simulink model "SimulinkModel_hquad_lin_roll_1stOrd"  (Simulink 7.6)
settings: Solver=ode45  StartTime=0.0  StopTime=10.0  RelTol=1e-3
values from neighbouring files (symbols this model uses):
  g = 9.8065    [kostas_malakies.mat]    (also in kostas_malakies2.mat; load_PMModel.m = 9.81; main.m; main_last.m)
  mass = 0.66    [kostas_malakies.mat]    (also in kostas_malakies2.mat; load_PMModel.m = 0.687; main_last.m)
libraries: Hqaud_model_LIB_SI x1
settings Model: Creator=andi  LastModifiedBy=burrimi
settings DebuggingCC: StrictBusMsg=Warning

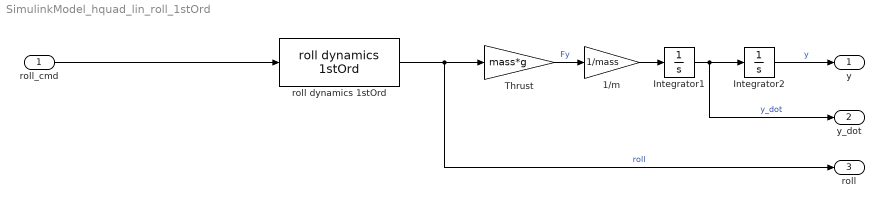
== system SimulinkModel_hquad_lin_roll_1stOrd ==
  roll_cmd : Inport
  1/m : Gain  Gain=1/mass
  Integrator1 : Integrator
  Integrator2 : Integrator
  Thrust : Gain  Gain=mass*g
  roll dynamics 1stOrd : Hqaud_model_LIB_SI/roll dynamics 1stOrd  SystemSampleTime=-1
  y : Outport
  y_dot : Outport  Port=2
  roll : Outport  Port=3
  wires:
  roll_cmd/1 -> roll dynamics 1stOrd/1
  Integrator2/1 -> y/1  "y"
  1/m/1 -> Integrator1/1
  roll dynamics 1stOrd/1 -> Thrust/1, roll/1  "roll"
  Integrator1/1 -> Integrator2/1, y_dot/1  "y_dot"
  Thrust/1 -> 1/m/1  "Fy"
